simulink model "PercobaanElinKu2"  (R2021a)
settings: Solver=VariableStepAuto  StartTime=0.0  StopTime=10.0  RelTol=1e-3
undefined symbols (not defined in the file or in its folder): kn
libraries: simulink x1
settings Model: Creator=asus  LastModifiedBy=asus

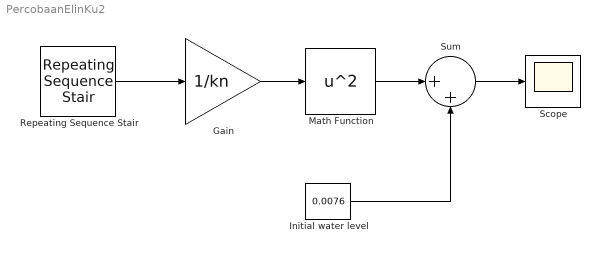
== system PercobaanElinKu2 ==
  Gain : Gain  Gain=1/kn
  Initial water level : Constant  Value=0.0076
  Math Function : Math  Operator=square  SaturateOnIntegerOverflow=on
  Repeating Sequence Stair : simulink/Sources/Repeating Sequence Stair  OutValues=[3 1 4 2 1].'  tsamp=-1  OutMin=[]  OutMax=[]  OutDataTypeStr=double  OutputDataTypeScalingMode=double  OutDataType=fixdt(0,8)  ConRadixGroup=Best Precision: Vector-wise  OutScaling=2^-12
  Scope : Scope
  Sum : Sum  Inputs=|++
  wires:
  Math Function/1 -> Sum/1
  Gain/1 -> Math Function/1
  Repeating Sequence Stair/1 -> Gain/1
  Sum/1 -> Scope/1
  Initial water level/1 -> Sum/2
